simulink model "ForwardDynamics_sim"  (Simulink 9.0)
settings: Solver=ode45  StartTime=0.0  StopTime=1  RelTol=1e-3  EnableMultiTasking=on
settings Model: Creator=gwu  LastModifiedBy=JayJay
settings DataIOCC: LimitDataPoints=on  SignalLoggingSaveFormat=ModelDataLogs
settings OptimizationCC: ExpressionDepthLimit=2147483647
settings DebuggingCC: SolverPrmCheckMsg=warning  FcnCallInpInsideContextMsg=warning  StateNameClashWarn=warning
settings RTWCC: TargetLang=C++
settings GRTTargetCC: GeneratePreprocessorConditionals=Disable all

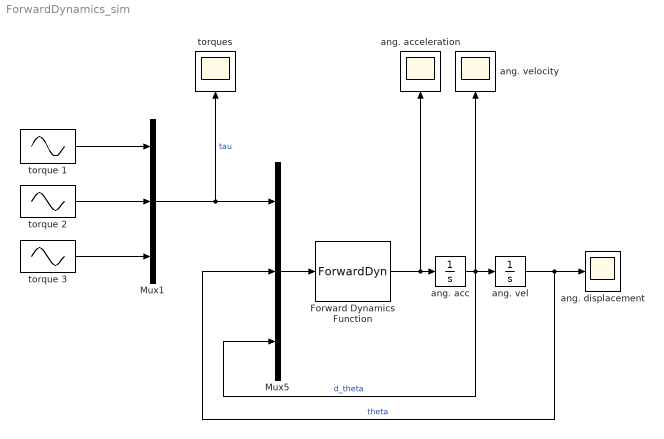
== system ForwardDynamics_sim ==
  Forward Dynamics Function : MATLABFcn  MATLABFcn=ForwardDyn  OutputDimensions=3
  Mux1 : Mux  Inputs=3
  Mux5 : Mux  Inputs=3
  ang. acc : Integrator
  ang. acceleration : Scope
  ang. displacement : Scope
  ang. vel : Integrator
  ang. velocity : Scope
  torque 1 : Sin  Amplitude=0  Frequency=2  SampleTime=0
  torque 2 : Sin  Amplitude=1.4  Frequency=2  SampleTime=0
  torque 3 : Sin  Amplitude=0.397  Frequency=2  SampleTime=0
  torques : Scope
  wires:
  ang. acc/1 -> ang. vel/1, Mux5/3, ang. velocity/1  "d_theta"
  Forward Dynamics Function/1 -> ang. acc/1, ang. acceleration/1
  Mux5/1 -> Forward Dynamics Function/1
  torque 2/1 -> Mux1/2
  torque 1/1 -> Mux1/1
  Mux1/1 -> Mux5/1, torques/1  "tau"
  ang. vel/1 -> ang. displacement/1, Mux5/2  "theta"
  torque 3/1 -> Mux1/3
